simulink model "sampleModel6"  (Simulink 9.1)
settings: Solver=VariableStepAuto  StartTime=0.0  StopTime=10.0  RelTol=1e-3
undefined symbols (not defined in the file): DiscIntNeverNeededParam, Newton, Raphson
libraries: simulink x14
settings Model: Creator=DELL  LastModifiedBy=DELL
settings DataIOCC: SaveFormat=Dataset
settings OptimizationCC: LifeSpan=auto
settings DebuggingCC: UnderspecifiedInitializationDetection=Simplified  MergeDetectMultiDrivingBlocksExec=error  SFUnexpectedBacktrackingDiag=error  SFNoUnconditionalDefaultTransitionDiag=error  SFExecutionAtInitializationDiag=warning
settings HardwareCC: ProdBitPerPointer=64  ProdBitPerSizeT=64  ProdBitPerPtrDiffT=64  ProdLargestAtomicFloat=Float  ProdIntDivRoundTo=Zero  ProdEndianess=LittleEndian  ProdWordSize=64  ProdHWDeviceType=Intel->x86-64 (Windows64)
settings ModelReferenceCC: PropagateSignalLabelsOutOfModel=on
settings CodeAppCC: StateflowObjectComments=off
settings GRTTargetCC: TargetLangStandard=C99 (ISO)  CombineOutputUpdateFcns=on  GRTInterface=off
settings ConfigComp: CovMetricSettings=dwe  CovHtmlReporting=off  CovSaveCumulativeToWorkspaceVar=off  CovSaveSingleToWorkspaceVar=off  CovExternalEMLEnable=on

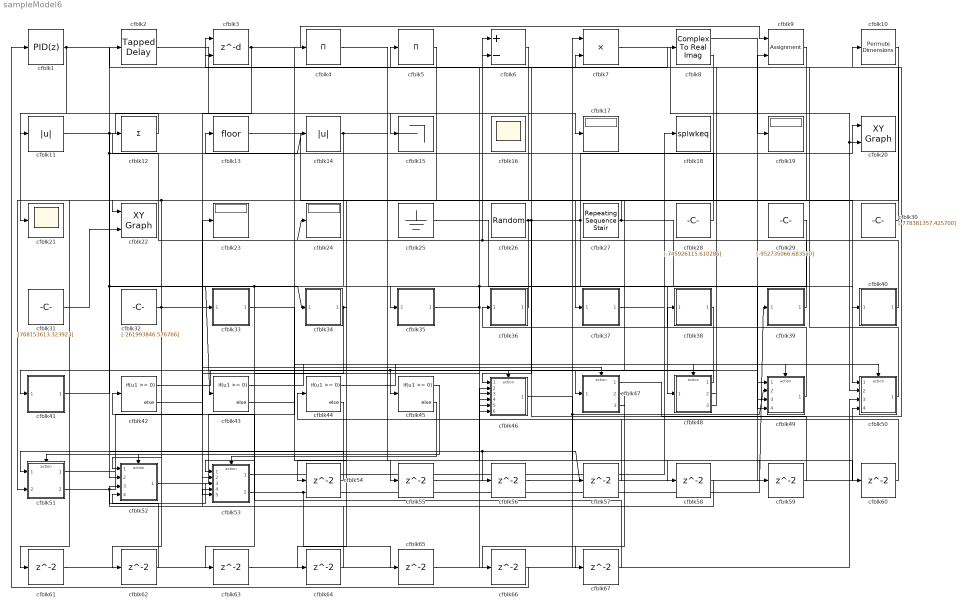
== system sampleModel6 ==
  cfblk1 : simulink/Continuous/PID Controller  Controller=PID  TimeDomain=Discrete-time  SampleTime=1  IntegratorMethod=Forward Euler  FilterMethod=Forward Euler  Form=Parallel  UseFilter=on  ControllerParametersSource=internal  P=1  I=1  D=0  N=100  InitialConditionSource=internal  InitialConditionForIntegrator=0  InitialConditionForFilter=0  ExternalReset=none  LimitOutput=off  UpperSaturationLimit=inf  LowerSaturationLimit=-inf  LinearizeAsGain=off  AntiWindupMode=none  Kb=1  TrackingMode=off  Kt=1  PParamMin=[]  PParamMax=[]  IParamMin=[]  IParamMax=[]  DParamMin=[]  DParamMax=[]  NParamMin=[]  NParamMax=[]  KbParamMin=[]  KbParamMax=[]  KtParamMin=[]  KtParamMax=[]  POutMin=[]  POutMax=[]  IOutMin=[]  IOutMax=[]  DOutMin=[]  DOutMax=[]  NOutMin=[]  NOutMax=[]  KbOutMin=[]  KbOutMax=[]  KtOutMin=[]  KtOutMax=[]  IntegratorOutMin=[]  IntegratorOutMax=[]  FilterOutMin=[]  FilterOutMax=[]  SumOutMin=[]  SumOutMax=[]  SumI1OutMin=[]  SumI1OutMax=[]  SumI2OutMin=[]  SumI2OutMax=[]  SumI3OutMin=[]  SumI3OutMax=[]  SumDOutMin=[]  SumDOutMax=[]  SaturationOutMin=[]  SaturationOutMax=[]  IntegratorContinuousStateAttributes=''  IntegratorStateMustResolveToSignalObject=off  IntegratorRTWStateStorageClass=Auto  FilterContinuousStateAttributes=''  FilterStateMustResolveToSignalObject=off  FilterRTWStateStorageClass=Auto  DifferentiatorICPrevScaledInput=0  DifferentiatorOutMin=[]  DifferentiatorOutMax=[]  FilterDiffOutCoefMin=[]  FilterDiffOutCoefMax=[]  SumDenOutMin=[]  SumDenOutMax=[]  SumNumOutMin=[]  SumNumOutMax=[]  ReciprocalOutMin=[]  ReciprocalOutMax=[]  DivideOutMin=[]  DivideOutMax=[]  TunerSelectOption=Transfer Function Based (PID Tuner App)
  cfblk10 : PermuteDimensions
  cfblk11 : Abs
  cfblk12 : Sum  Inputs=+
  cfblk13 : Rounding
  cfblk14 : Abs
  cfblk15 : Terminator
  cfblk16 : Scope
      settings: Floating=on
  cfblk{17,19,23..24} (4 alike) : Display
  cfblk18 : ToWorkspace  VariableName=splwkeq  SaveFormat=Timeseries  SampleTime=-1
  cfblk2 : simulink/Discrete/Tapped Delay  vinit=0.0  samptime=-1  NumDelays=1  DelayOrder=Oldest  includeCurrent=off
  cfblk20 : simulink/Sinks/XY Graph  xmin=-1  xmax=1  ymin=-1  ymax=1  st=-1
  cfblk21 : Scope
  cfblk22 : simulink/Sinks/XY Graph  xmin=-1  xmax=1  ymin=-1  ymax=1  st=-1
  cfblk25 : Ground
  cfblk26 : UniformRandomNumber  Minimum=[-3759994456.876560]  Maximum=[3279415969.732488]  Seed=[80296531.000000]  SampleTime=0.1
  cfblk27 : simulink/Sources/Repeating Sequence Stair  OutValues=[998955717.271784, 961956321.864293]  tsamp=-1  OutMin=[]  OutMax=[]  OutDataTypeStr=double  OutputDataTypeScalingMode=double  OutDataType=fixdt(0,8)  ConRadixGroup=Best Precision: Vector-wise  OutScaling=2^-12
  cfblk28 : Constant  Value=[-745926115.610286]  SampleTime=1
  cfblk29 : Constant  Value=[-952735066.683550]  SampleTime=1
  cfblk3 : Delay  DelayLengthSource=Input port  SampleTime=1
      settings: InputPortMap=u0,p1
  cfblk30 : Constant  Value=[-778381357.425700]  SampleTime=1
  cfblk31 : Constant  Value=[768153613.323923]  SampleTime=1
  cfblk32 : Constant  Value=[-261993846.576766]  SampleTime=1
  cfblk33 : Subsystem
  cfblk34 : Subsystem
  cfblk35 : Subsystem
  cfblk36 : Subsystem
  cfblk37 : Subsystem
  cfblk38 : Subsystem
  cfblk39 : Subsystem
  cfblk4 : Product  Inputs=*
  cfblk40 : Subsystem
  cfblk41 : Subsystem
  cfblk{42..45} (4 alike) : If  IfExpression=u1 >= 0  SampleTime=1
  cfblk46 : Subsystem  TreatAsAtomicUnit=on
  cfblk47 : Subsystem  TreatAsAtomicUnit=on
  cfblk48 : Subsystem  TreatAsAtomicUnit=on
  cfblk49 : Subsystem  TreatAsAtomicUnit=on
  cfblk5 : Product  Inputs=*
  cfblk50 : Subsystem  TreatAsAtomicUnit=on
  cfblk51 : Subsystem  TreatAsAtomicUnit=on
  cfblk52 : Subsystem  TreatAsAtomicUnit=on
  cfblk53 : Subsystem  TreatAsAtomicUnit=on
  cfblk{54..67} (14 alike) : Delay  SampleTime=1
  cfblk6 : Sum  Inputs=+-
  cfblk7 : Product  Inputs=**
  cfblk8 : ComplexToRealImag
  cfblk9 : Assignment  DiagnosticForDimensions=Warning  IndexOptions=Index vector (dialog)  Indices=1  OutputSizes=1
  wires:
  cfblk28/1 -> cfblk13/1
  cfblk49/1(cfblk2) -> cfblk36/1(cfblk1)
  cfblk27/1 -> cfblk22/1, cfblk49/4(cfblk9)
  cfblk29/1 -> cfblk43/1, cfblk46/5(cfblk12)
  cfblk26/1 -> cfblk48/1(cfblk1), cfblk20/1, cfblk46/1(cfblk1), cfblk46/6(cfblk13)
  cfblk31/1 -> cfblk22/2
  cfblk3/1 -> cfblk9/1, cfblk53/5(cfblk10)
  cfblk50/1(cfblk2) -> cfblk3/1
  cfblk47/1(cfblk2) -> cfblk10/1
  cfblk48/1(cfblk2) -> cfblk41/1(cfblk1)
  cfblk53/1(cfblk2) -> cfblk18/1
  cfblk48/2(cfblk8) -> cfblk38/1(cfblk1)
  cfblk1/1 -> cfblk21/1, cfblk7/2
  cfblk10/1 -> cfblk37/1(cfblk1)
  cfblk40/1(cfblk2) -> cfblk24/1, cfblk6/2
  cfblk36/1(cfblk2) -> cfblk35/1(cfblk1)
  cfblk11/1 -> cfblk56/1, cfblk57/1, cfblk34/1(cfblk1), cfblk17/1
  cfblk2/1 -> cfblk15/1
  cfblk53/2(cfblk11) -> cfblk39/1(cfblk1), cfblk65/1
  cfblk13/1 -> cfblk50/1(cfblk1)
  cfblk48/3(cfblk9) -> cfblk6/1
  cfblk30/1 -> cfblk5/1
  cfblk37/1(cfblk2) -> cfblk40/1(cfblk1)
  cfblk38/1(cfblk2) -> cfblk45/1, cfblk53/2(cfblk7)
  cfblk8/1 -> cfblk19/1
  cfblk9/1 -> cfblk47/1(cfblk1)
  cfblk52/1(cfblk2) -> cfblk4/1
  cfblk41/1(cfblk2) -> cfblk2/1, cfblk14/1
  cfblk5/1 -> cfblk51/2(cfblk14)
  cfblk51/1(cfblk2) -> cfblk33/1(cfblk1)
  cfblk39/1(cfblk2) -> cfblk12/1
  cfblk35/1(cfblk2) -> cfblk8/1, cfblk60/1
  cfblk7/1 -> cfblk50/2(cfblk10), cfblk20/2
  cfblk51/2(cfblk15) -> cfblk23/1, cfblk53/3(cfblk8)
  cfblk25/1 -> cfblk49/1(cfblk1)
  cfblk12/1 -> cfblk11/1
  cfblk32/1 -> cfblk52/1(cfblk1), cfblk46/3(cfblk10)
  cfblk8/2 -> cfblk61/1, cfblk62/1
  cfblk14/1 -> cfblk52/2(cfblk13), cfblk53/1(cfblk1), cfblk49/3(cfblk8)
  cfblk46/1(cfblk2) -> cfblk49/2(cfblk7), cfblk58/1
  cfblk34/1(cfblk2) -> cfblk63/1, cfblk64/1
  cfblk42/1 -> cfblk46/Action
  cfblk42/2 -> cfblk47/Action
  cfblk43/1 -> cfblk48/Action
  cfblk43/2 -> cfblk49/Action
  cfblk44/1 -> cfblk50/Action
  cfblk44/2 -> cfblk51/Action
  cfblk45/1 -> cfblk52/Action
  cfblk45/2 -> cfblk53/Action
  cfblk6/1 -> cfblk54/1
  cfblk54/1 -> cfblk51/1(cfblk1)
  cfblk33/1(cfblk2) -> cfblk55/1
  cfblk55/1 -> cfblk9/2
  cfblk56/1 -> cfblk50/4(cfblk12)
  cfblk57/1 -> cfblk46/2(cfblk9)
  cfblk58/1 -> cfblk52/3(cfblk14)
  cfblk4/1 -> cfblk59/1
  cfblk59/1 -> cfblk3/2
  cfblk60/1 -> cfblk44/1
  cfblk61/1 -> cfblk50/3(cfblk11)
  cfblk62/1 -> cfblk52/4(cfblk15)
  cfblk63/1 -> cfblk7/1
  cfblk64/1 -> cfblk53/4(cfblk9)
  cfblk65/1 -> cfblk46/4(cfblk11)
  cfblk47/2(cfblk13) -> cfblk66/1
  cfblk66/1 -> cfblk1/1
  cfblk47/3(cfblk14) -> cfblk67/1
  cfblk67/1 -> cfblk42/1

== system sampleModel6/cfblk33 ==
  cfblk1 : Inport
  cfblk2 : Outport
  wires:
  cfblk1/1 -> cfblk2/1

== system sampleModel6/cfblk34 ==
  cfblk1 : Inport
  cfblk2 : Outport
  wires:
  cfblk1/1 -> cfblk2/1

== system sampleModel6/cfblk35 ==
  cfblk1 : Inport
  cfblk2 : Outport
  wires:
  cfblk1/1 -> cfblk2/1

== system sampleModel6/cfblk36 ==
  cfblk1 : Inport
  cfblk2 : Outport
  wires:
  cfblk1/1 -> cfblk2/1

== system sampleModel6/cfblk37 ==
  cfblk1 : Inport
  cfblk2 : Outport
  wires:
  cfblk1/1 -> cfblk2/1

== system sampleModel6/cfblk38 ==
  cfblk1 : Inport
  cfblk2 : Outport
  wires:
  cfblk1/1 -> cfblk2/1

== system sampleModel6/cfblk39 ==
  cfblk1 : Inport
  cfblk2 : Outport
  wires:
  cfblk1/1 -> cfblk2/1

== system sampleModel6/cfblk40 ==
  cfblk1 : Inport
  cfblk2 : Outport
  wires:
  cfblk1/1 -> cfblk2/1

== system sampleModel6/cfblk41 ==
  cfblk1 : Inport
  cfblk2 : Outport
  wires:
  cfblk1/1 -> cfblk2/1

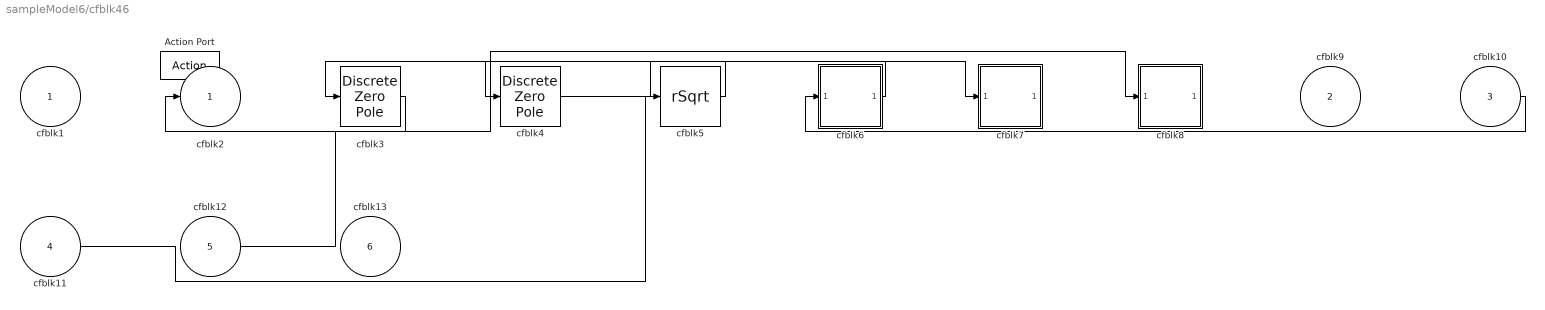
== system sampleModel6/cfblk46 ==
  cfblk1 : Inport
  cfblk9 : Inport  Port=2
  cfblk10 : Inport  Port=3
  cfblk11 : Inport  Port=4
  cfblk12 : Inport  Port=5
  cfblk13 : Inport  Port=6
  Action Port : ActionPort  ActionType=then
  cfblk3 : DiscreteZeroPole  Poles=[0 0.5]  Gain=1  SampleTime=-1
  cfblk4 : DiscreteZeroPole  Poles=[0 0.5]  Gain=1  SampleTime=-1
  cfblk5 : Sqrt  Operator=rSqrt  AlgorithmType=Newton-Raphson  SaturateOnIntegerOverflow=on
  cfblk6 : Subsystem
  cfblk7 : Subsystem
  cfblk8 : Subsystem
  cfblk2 : Outport
  wires:
  cfblk4/1 -> cfblk7/1(cfblk1)
  cfblk10/1 -> cfblk6/1(cfblk1)
  cfblk12/1 -> cfblk8/1(cfblk1)
  cfblk6/1(cfblk2) -> cfblk3/1
  cfblk5/1 -> cfblk4/1
  cfblk11/1 -> cfblk5/1
  cfblk3/1 -> cfblk2/1

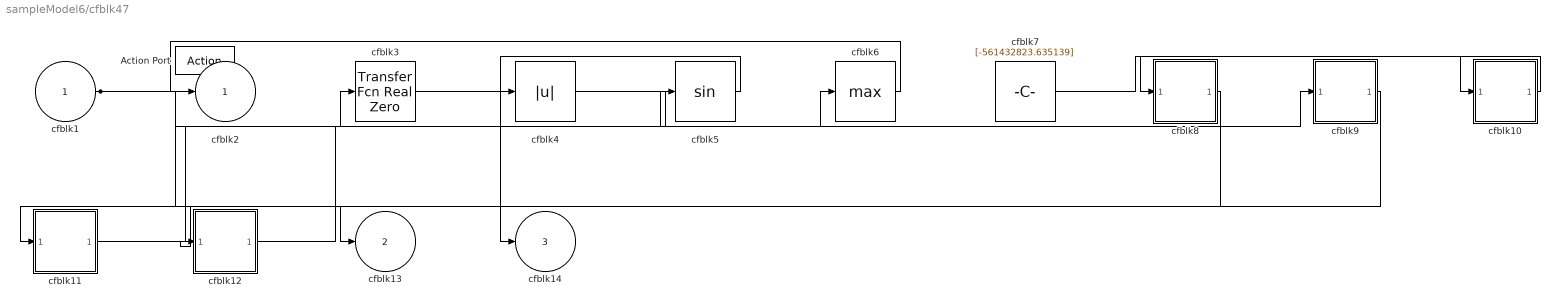
== system sampleModel6/cfblk47 ==
  cfblk1 : Inport
  Action Port : ActionPort  ActionType=else
  cfblk10 : Subsystem
  cfblk11 : Subsystem
  cfblk12 : Subsystem
  cfblk3 : simulink/Discrete/Transfer Fcn Real Zero  ZeroZ=0.75  ICPrevInput=0.0  DoSatur=off
      settings: SourceProductName=Simulink  SourceProductBaseCode=SL
  cfblk4 : Abs
  cfblk5 : Trigonometry
  cfblk6 : MinMax  Function=max
  cfblk7 : Constant  Value=[-561432823.635139]  SampleTime=1
  cfblk8 : Subsystem
  cfblk9 : Subsystem
  cfblk2 : Outport
  cfblk13 : Outport  Port=2
  cfblk14 : Outport  Port=3
  wires:
  cfblk11/1(cfblk2) -> cfblk3/1
  cfblk6/1 -> cfblk2/1
  cfblk9/1(cfblk2) -> cfblk12/1(cfblk1)
  cfblk10/1(cfblk2) -> cfblk8/1(cfblk1)
  cfblk3/1 -> cfblk14/1
  cfblk5/1 -> cfblk4/1
  cfblk4/1 -> cfblk9/1(cfblk1)
  cfblk1/1 -> cfblk13/1, cfblk5/1
  cfblk7/1 -> cfblk10/1(cfblk1)
  cfblk8/1(cfblk2) -> cfblk11/1(cfblk1)
  cfblk12/1(cfblk2) -> cfblk6/1

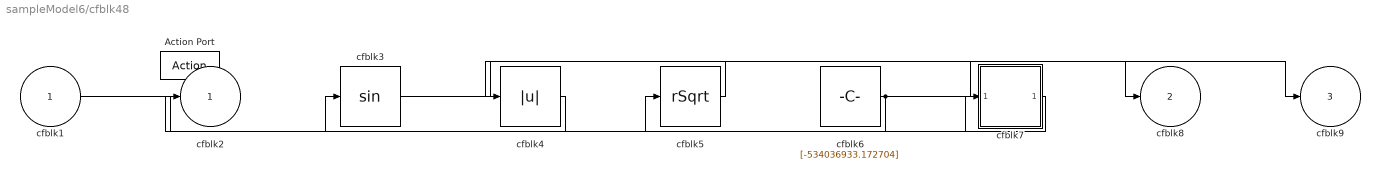
== system sampleModel6/cfblk48 ==
  cfblk1 : Inport
  Action Port : ActionPort  ActionType=then
  cfblk3 : Trigonometry
  cfblk4 : Abs
  cfblk5 : Sqrt  Operator=rSqrt  AlgorithmType=Newton-Raphson  SaturateOnIntegerOverflow=on
  cfblk6 : Constant  Value=[-534036933.172704]  SampleTime=1
  cfblk7 : Subsystem
  cfblk2 : Outport
  cfblk8 : Outport  Port=2
  cfblk9 : Outport  Port=3
  wires:
  cfblk3/1 -> cfblk8/1
  cfblk4/1 -> cfblk3/1
  cfblk7/1(cfblk2) -> cfblk5/1
  cfblk5/1 -> cfblk4/1
  cfblk6/1 -> cfblk9/1, cfblk2/1
  cfblk1/1 -> cfblk7/1(cfblk1)

== system sampleModel6/cfblk49 ==
  cfblk1 : Inport
  cfblk7 : Inport  Port=2
  cfblk8 : Inport  Port=3
  cfblk9 : Inport  Port=4
  Action Port : ActionPort  ActionType=else
  cfblk3 : simulink/Continuous/PID Controller  Controller=PID  TimeDomain=Discrete-time  SampleTime=-1  IntegratorMethod=Forward Euler  FilterMethod=Forward Euler  Form=Parallel  UseFilter=on  ControllerParametersSource=internal  P=1  I=1  D=0  N=100  InitialConditionSource=internal  InitialConditionForIntegrator=0  InitialConditionForFilter=0  ExternalReset=none  LimitOutput=off  UpperSaturationLimit=inf  LowerSaturationLimit=-inf  LinearizeAsGain=off  AntiWindupMode=none  Kb=1  TrackingMode=off  Kt=1  PParamMin=[]  PParamMax=[]  IParamMin=[]  IParamMax=[]  DParamMin=[]  DParamMax=[]  NParamMin=[]  NParamMax=[]  KbParamMin=[]  KbParamMax=[]  KtParamMin=[]  KtParamMax=[]  POutMin=[]  POutMax=[]  IOutMin=[]  IOutMax=[]  DOutMin=[]  DOutMax=[]  NOutMin=[]  NOutMax=[]  KbOutMin=[]  KbOutMax=[]  KtOutMin=[]  KtOutMax=[]  IntegratorOutMin=[]  IntegratorOutMax=[]  FilterOutMin=[]  FilterOutMax=[]  SumOutMin=[]  SumOutMax=[]  SumI1OutMin=[]  SumI1OutMax=[]  SumI2OutMin=[]  SumI2OutMax=[]  SumI3OutMin=[]  SumI3OutMax=[]  SumDOutMin=[]  SumDOutMax=[]  SaturationOutMin=[]  SaturationOutMax=[]  IntegratorContinuousStateAttributes=''  IntegratorStateMustResolveToSignalObject=off  IntegratorRTWStateStorageClass=Auto  FilterContinuousStateAttributes=''  FilterStateMustResolveToSignalObject=off  FilterRTWStateStorageClass=Auto  DifferentiatorICPrevScaledInput=0  DifferentiatorOutMin=[]  DifferentiatorOutMax=[]  FilterDiffOutCoefMin=[]  FilterDiffOutCoefMax=[]  SumDenOutMin=[]  SumDenOutMax=[]  SumNumOutMin=[]  SumNumOutMax=[]  ReciprocalOutMin=[]  ReciprocalOutMax=[]  DivideOutMin=[]  DivideOutMax=[]  TunerSelectOption=Transfer Function Based (PID Tuner App)
  cfblk4 : simulink/Math Operations/MinMax Running Resettable  Function=min  vinit=0.0
  cfblk5 : Constant  Value=[144478436.825369]  SampleTime=1
  cfblk6 : Subsystem
  cfblk2 : Outport
  wires:
  cfblk9/1 -> cfblk3/1
  cfblk8/1 -> cfblk4/1
  cfblk5/1 -> cfblk2/1
  cfblk7/1 -> cfblk6/1(cfblk1)
  cfblk3/1 -> cfblk4/2

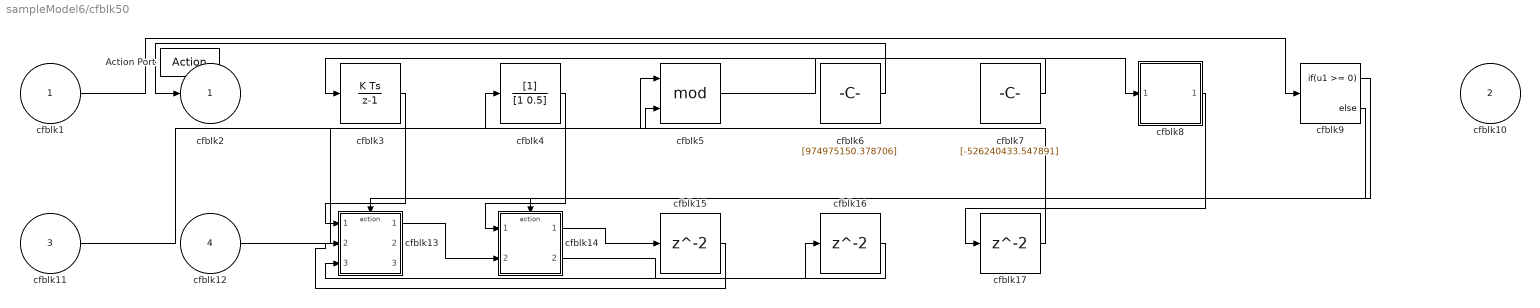
== system sampleModel6/cfblk50 ==
  cfblk1 : Inport
  cfblk10 : Inport  Port=2
  cfblk11 : Inport  Port=3
  cfblk12 : Inport  Port=4
  Action Port : ActionPort  ActionType=then
  cfblk13 : Subsystem  TreatAsAtomicUnit=on
  cfblk14 : Subsystem  TreatAsAtomicUnit=on
  cfblk15 : Delay
  cfblk16 : Delay
  cfblk17 : Delay
  cfblk3 : DiscreteIntegrator  SampleTime=-1  ICPrevOutput=DiscIntNeverNeededParam  ICPrevScaledInput=DiscIntNeverNeededParam
  cfblk4 : DiscreteFilter
  cfblk5 : Math  Operator=mod  SaturateOnIntegerOverflow=on
  cfblk6 : Constant  Value=[974975150.378706]  SampleTime=1
  cfblk7 : Constant  Value=[-526240433.547891]  SampleTime=1
  cfblk8 : Subsystem
  cfblk9 : If  IfExpression=u1 >= 0  SampleTime=1
  cfblk2 : Outport
  wires:
  cfblk4/1 -> cfblk14/1(cfblk1)
  cfblk6/1 -> cfblk2/1
  cfblk12/1 -> cfblk5/2
  cfblk7/1 -> cfblk3/1
  cfblk5/1 -> cfblk8/1(cfblk1)
  cfblk11/1 -> cfblk4/1
  cfblk1/1 -> cfblk9/1
  cfblk3/1 -> cfblk13/1(cfblk1)
  cfblk13/1(cfblk2) -> cfblk14/2(cfblk14)
  cfblk9/1 -> cfblk13/Action
  cfblk9/2 -> cfblk14/Action
  cfblk14/1(cfblk2) -> cfblk15/1
  cfblk15/1 -> cfblk13/2(cfblk13)
  cfblk14/2(cfblk15) -> cfblk16/1
  cfblk16/1 -> cfblk13/3(cfblk14)
  cfblk8/1(cfblk2) -> cfblk17/1
  cfblk17/1 -> cfblk5/1

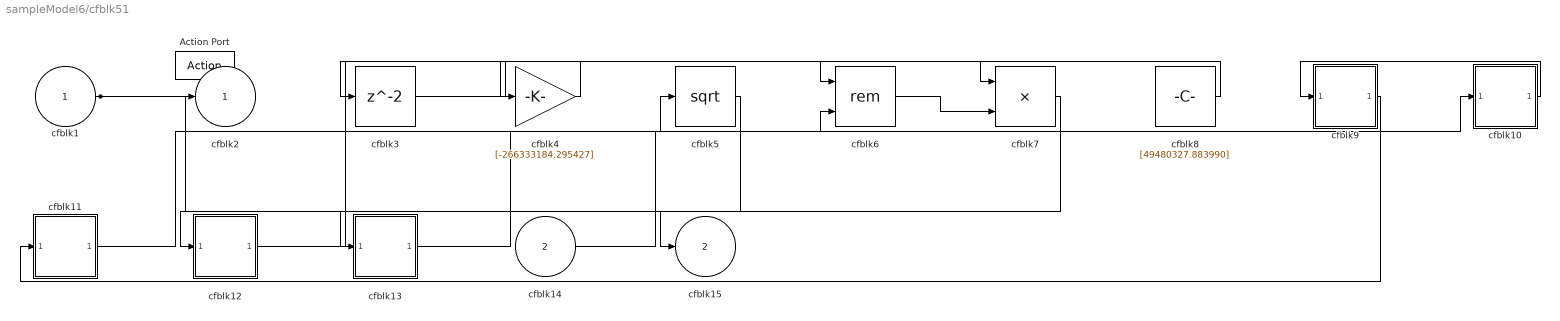
== system sampleModel6/cfblk51 ==
  cfblk1 : Inport
  cfblk14 : Inport  Port=2
  Action Port : ActionPort  ActionType=else
  cfblk10 : Subsystem
  cfblk11 : Subsystem
  cfblk12 : Subsystem
  cfblk13 : Subsystem
  cfblk3 : Delay
  cfblk4 : Gain  Gain=[-266333184.295427]
  cfblk5 : Sqrt  SaturateOnIntegerOverflow=on
  cfblk6 : Math  Operator=rem  SaturateOnIntegerOverflow=on
  cfblk7 : Product
  cfblk8 : Constant  Value=[49480327.883990]  SampleTime=1
  cfblk9 : Subsystem
  cfblk2 : Outport
  cfblk15 : Outport  Port=2
  wires:
  cfblk13/1(cfblk2) -> cfblk5/1
  cfblk12/1(cfblk2) -> cfblk7/1
  cfblk4/1 -> cfblk3/1
  cfblk1/1 -> cfblk13/1(cfblk1), cfblk2/1
  cfblk9/1(cfblk2) -> cfblk11/1(cfblk1)
  cfblk6/1 -> cfblk7/2
  cfblk7/1 -> cfblk15/1
  cfblk3/1 -> cfblk6/1
  cfblk8/1 -> cfblk4/1
  cfblk5/1 -> cfblk12/1(cfblk1)
  cfblk11/1(cfblk2) -> cfblk6/2
  cfblk14/1 -> cfblk10/1(cfblk1)
  cfblk10/1(cfblk2) -> cfblk9/1(cfblk1)

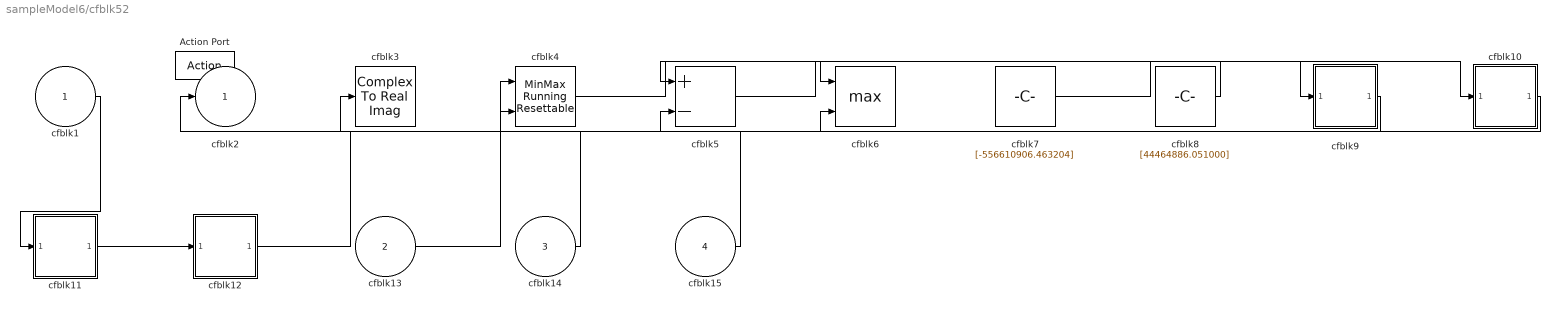
== system sampleModel6/cfblk52 ==
  cfblk1 : Inport
  cfblk13 : Inport  Port=2
  cfblk14 : Inport  Port=3
  cfblk15 : Inport  Port=4
  Action Port : ActionPort  ActionType=then
  cfblk10 : Subsystem
  cfblk11 : Subsystem
  cfblk12 : Subsystem
  cfblk3 : ComplexToRealImag
  cfblk4 : simulink/Math Operations/MinMax Running Resettable  Function=min  vinit=0.0
  cfblk5 : Sum  Inputs=+-
  cfblk6 : MinMax  Function=max  Inputs=2
  cfblk7 : Constant  Value=[-556610906.463204]  SampleTime=1
  cfblk8 : Constant  Value=[44464886.051000]  SampleTime=1
  cfblk9 : Subsystem
  cfblk2 : Outport
  wires:
  cfblk7/1 -> cfblk10/1(cfblk1)
  cfblk10/1(cfblk2) -> cfblk2/1
  cfblk13/1 -> cfblk4/1
  cfblk4/1 -> cfblk6/1
  cfblk11/1(cfblk2) -> cfblk12/1(cfblk1)
  cfblk1/1 -> cfblk11/1(cfblk1)
  cfblk14/1 -> cfblk3/1
  cfblk12/1(cfblk2) -> cfblk6/2
  cfblk8/1 -> cfblk5/1
  cfblk15/1 -> cfblk5/2
  cfblk5/1 -> cfblk9/1(cfblk1)
  cfblk9/1(cfblk2) -> cfblk4/2

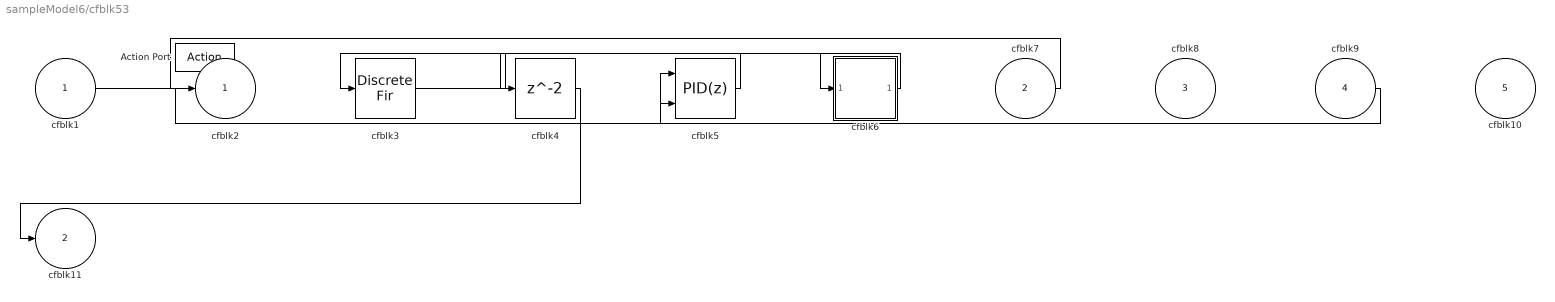
== system sampleModel6/cfblk53 ==
  cfblk1 : Inport
  cfblk7 : Inport  Port=2
  cfblk8 : Inport  Port=3
  cfblk9 : Inport  Port=4
  cfblk10 : Inport  Port=5
  Action Port : ActionPort  ActionType=else
  cfblk3 : DiscreteFir
  cfblk4 : Delay
  cfblk5 : simulink/Continuous/PID Controller (2DOF)  Controller=PID  TimeDomain=Discrete-time  SampleTime=-1  IntegratorMethod=Forward Euler  FilterMethod=Forward Euler  Form=Parallel  UseFilter=on  ControllerParametersSource=internal  P=1  I=1  D=0  N=100  b=1  c=1  InitialConditionSource=internal  InitialConditionForIntegrator=0  InitialConditionForFilter=0  ExternalReset=none  LimitOutput=off  UpperSaturationLimit=inf  LowerSaturationLimit=-inf  LinearizeAsGain=off  AntiWindupMode=none  Kb=1  TrackingMode=off  Kt=1  PParamMin=[]  PParamMax=[]  IParamMin=[]  IParamMax=[]  DParamMin=[]  DParamMax=[]  NParamMin=[]  NParamMax=[]  bParamMin=[]  bParamMax=[]  cParamMin=[]  cParamMax=[]  KbParamMin=[]  KbParamMax=[]  KtParamMin=[]  KtParamMax=[]  POutMin=[]  POutMax=[]  IOutMin=[]  IOutMax=[]  DOutMin=[]  DOutMax=[]  NOutMin=[]  NOutMax=[]  bOutMin=[]  bOutMax=[]  cOutMin=[]  cOutMax=[]  KbOutMin=[]  KbOutMax=[]  KtOutMin=[]  KtOutMax=[]  IntegratorOutMin=[]  IntegratorOutMax=[]  FilterOutMin=[]  FilterOutMax=[]  SumOutMin=[]  SumOutMax=[]  Sum1OutMin=[]  Sum1OutMax=[]  Sum2OutMin=[]  Sum2OutMax=[]  Sum3OutMin=[]  Sum3OutMax=[]  SumI1OutMin=[]  SumI1OutMax=[]  SumI2OutMin=[]  SumI2OutMax=[]  SumI3OutMin=[]  SumI3OutMax=[]  SumDOutMin=[]  SumDOutMax=[]  SaturationOutMin=[]  SaturationOutMax=[]  IntegratorContinuousStateAttributes=''  IntegratorStateMustResolveToSignalObject=off  IntegratorRTWStateStorageClass=Auto  FilterContinuousStateAttributes=''  FilterStateMustResolveToSignalObject=off  FilterRTWStateStorageClass=Auto  DifferentiatorICPrevScaledInput=0  DifferentiatorOutMin=[]  DifferentiatorOutMax=[]  FilterDiffOutCoefMin=[]  FilterDiffOutCoefMax=[]  SumDenOutMin=[]  SumDenOutMax=[]  SumNumOutMin=[]  SumNumOutMax=[]  ReciprocalOutMin=[]  ReciprocalOutMax=[]  DivideOutMin=[]  DivideOutMax=[]  TunerSelectOption=Transfer Function Based (PID Tuner App)
  cfblk6 : Subsystem
  cfblk2 : Outport
  cfblk11 : Outport  Port=2
  wires:
  cfblk5/1 -> cfblk3/1
  cfblk4/1 -> cfblk11/1
  cfblk7/1 -> cfblk2/1
  cfblk3/1 -> cfblk6/1(cfblk1)
  cfblk9/1 -> cfblk5/1
  cfblk6/1(cfblk2) -> cfblk4/1
  cfblk1/1 -> cfblk5/2

== system sampleModel6/cfblk46/cfblk6 ==
  cfblk1 : Inport
  cfblk2 : Outport
  wires:
  cfblk1/1 -> cfblk2/1

== system sampleModel6/cfblk46/cfblk7 ==
  cfblk1 : Inport
  cfblk2 : Outport
  wires:
  cfblk1/1 -> cfblk2/1

== system sampleModel6/cfblk46/cfblk8 ==
  cfblk1 : Inport
  cfblk2 : Outport
  wires:
  cfblk1/1 -> cfblk2/1

== system sampleModel6/cfblk47/cfblk10 ==
  cfblk1 : Inport
  cfblk2 : Outport
  wires:
  cfblk1/1 -> cfblk2/1

== system sampleModel6/cfblk47/cfblk11 ==
  cfblk1 : Inport
  cfblk2 : Outport
  wires:
  cfblk1/1 -> cfblk2/1

== system sampleModel6/cfblk47/cfblk12 ==
  cfblk1 : Inport
  cfblk2 : Outport
  wires:
  cfblk1/1 -> cfblk2/1

== system sampleModel6/cfblk47/cfblk8 ==
  cfblk1 : Inport
  cfblk2 : Outport
  wires:
  cfblk1/1 -> cfblk2/1

== system sampleModel6/cfblk47/cfblk9 ==
  cfblk1 : Inport
  cfblk2 : Outport
  wires:
  cfblk1/1 -> cfblk2/1

== system sampleModel6/cfblk48/cfblk7 ==
  cfblk1 : Inport
  cfblk2 : Outport
  wires:
  cfblk1/1 -> cfblk2/1

== system sampleModel6/cfblk49/cfblk6 ==
  cfblk1 : Inport
  cfblk2 : Outport
  wires:
  cfblk1/1 -> cfblk2/1

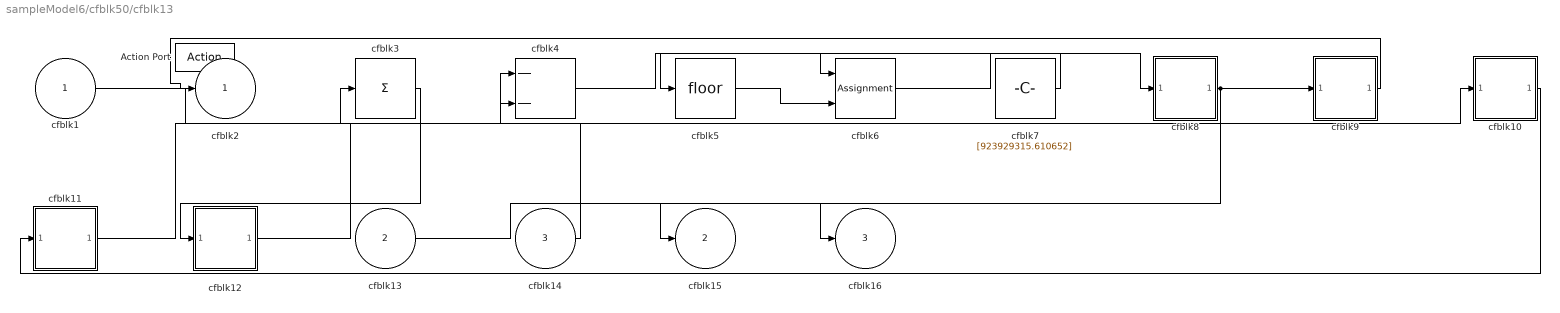
== system sampleModel6/cfblk50/cfblk13 ==
  cfblk1 : Inport
  cfblk13 : Inport  Port=2
  cfblk14 : Inport  Port=3
  Action Port : ActionPort  ActionType=then
  cfblk10 : Subsystem
  cfblk11 : Subsystem
  cfblk12 : Subsystem
  cfblk3 : Sum  Inputs=+
  cfblk4 : Sum  Inputs=--
  cfblk5 : Rounding
  cfblk6 : Assignment  DiagnosticForDimensions=Warning  IndexOptions=Index vector (dialog)  Indices=1  OutputSizes=1
  cfblk7 : Constant  Value=[923929315.610652]  SampleTime=1
  cfblk8 : Subsystem
  cfblk9 : Subsystem
  cfblk2 : Outport
  cfblk15 : Outport  Port=2
  cfblk16 : Outport  Port=3
  wires:
  cfblk1/1 -> cfblk10/1(cfblk1)
  cfblk7/1 -> cfblk5/1
  cfblk8/1(cfblk2) -> cfblk15/1, cfblk9/1(cfblk1)
  cfblk10/1(cfblk2) -> cfblk11/1(cfblk1)
  cfblk3/1 -> cfblk12/1(cfblk1)
  cfblk13/1 -> cfblk16/1
  cfblk9/1(cfblk2) -> cfblk2/1
  cfblk12/1(cfblk2) -> cfblk4/1
  cfblk11/1(cfblk2) -> cfblk4/2
  cfblk6/1 -> cfblk8/1(cfblk1)
  cfblk4/1 -> cfblk6/1
  cfblk5/1 -> cfblk6/2
  cfblk14/1 -> cfblk3/1

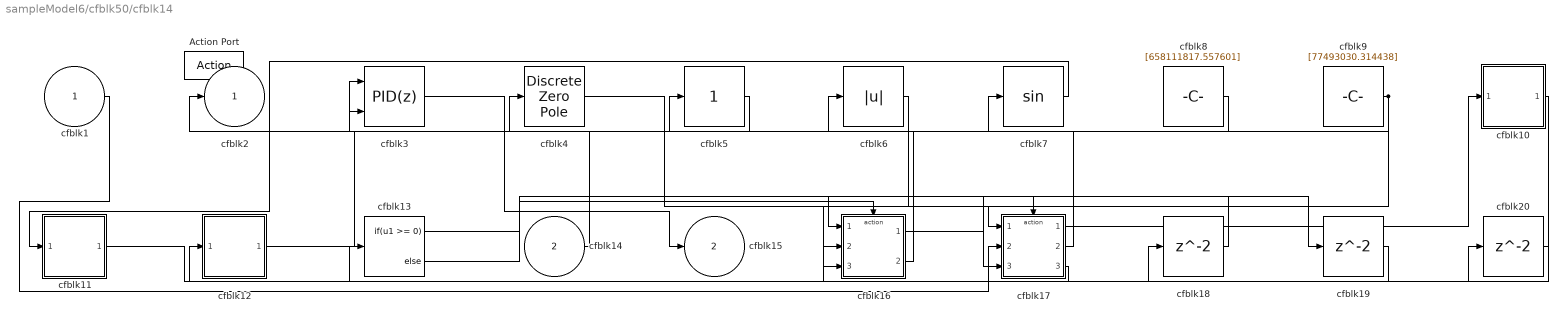
== system sampleModel6/cfblk50/cfblk14 ==
  cfblk1 : Inport
  cfblk14 : Inport  Port=2
  Action Port : ActionPort  ActionType=else
  cfblk10 : Subsystem
  cfblk11 : Subsystem
  cfblk12 : Subsystem
  cfblk13 : If  IfExpression=u1 >= 0  SampleTime=1
  cfblk16 : Subsystem  TreatAsAtomicUnit=on
  cfblk17 : Subsystem  TreatAsAtomicUnit=on
  cfblk18 : Delay
  cfblk19 : Delay
  cfblk20 : Delay
  cfblk3 : simulink/Continuous/PID Controller (2DOF)  Controller=PID  TimeDomain=Discrete-time  SampleTime=-1  IntegratorMethod=Forward Euler  FilterMethod=Forward Euler  Form=Parallel  UseFilter=on  ControllerParametersSource=internal  P=1  I=1  D=0  N=100  b=1  c=1  InitialConditionSource=internal  InitialConditionForIntegrator=0  InitialConditionForFilter=0  ExternalReset=none  LimitOutput=off  UpperSaturationLimit=inf  LowerSaturationLimit=-inf  LinearizeAsGain=off  AntiWindupMode=none  Kb=1  TrackingMode=off  Kt=1  PParamMin=[]  PParamMax=[]  IParamMin=[]  IParamMax=[]  DParamMin=[]  DParamMax=[]  NParamMin=[]  NParamMax=[]  bParamMin=[]  bParamMax=[]  cParamMin=[]  cParamMax=[]  KbParamMin=[]  KbParamMax=[]  KtParamMin=[]  KtParamMax=[]  POutMin=[]  POutMax=[]  IOutMin=[]  IOutMax=[]  DOutMin=[]  DOutMax=[]  NOutMin=[]  NOutMax=[]  bOutMin=[]  bOutMax=[]  cOutMin=[]  cOutMax=[]  KbOutMin=[]  KbOutMax=[]  KtOutMin=[]  KtOutMax=[]  IntegratorOutMin=[]  IntegratorOutMax=[]  FilterOutMin=[]  FilterOutMax=[]  SumOutMin=[]  SumOutMax=[]  Sum1OutMin=[]  Sum1OutMax=[]  Sum2OutMin=[]  Sum2OutMax=[]  Sum3OutMin=[]  Sum3OutMax=[]  SumI1OutMin=[]  SumI1OutMax=[]  SumI2OutMin=[]  SumI2OutMax=[]  SumI3OutMin=[]  SumI3OutMax=[]  SumDOutMin=[]  SumDOutMax=[]  SaturationOutMin=[]  SaturationOutMax=[]  IntegratorContinuousStateAttributes=''  IntegratorStateMustResolveToSignalObject=off  IntegratorRTWStateStorageClass=Auto  FilterContinuousStateAttributes=''  FilterStateMustResolveToSignalObject=off  FilterRTWStateStorageClass=Auto  DifferentiatorICPrevScaledInput=0  DifferentiatorOutMin=[]  DifferentiatorOutMax=[]  FilterDiffOutCoefMin=[]  FilterDiffOutCoefMax=[]  SumDenOutMin=[]  SumDenOutMax=[]  SumNumOutMin=[]  SumNumOutMax=[]  ReciprocalOutMin=[]  ReciprocalOutMax=[]  DivideOutMin=[]  DivideOutMax=[]  TunerSelectOption=Transfer Function Based (PID Tuner App)
  cfblk4 : DiscreteZeroPole  Poles=[0 0.5]  Gain=1  SampleTime=-1
  cfblk5 : simulink/Math Operations/Slider Gain  gain=1  low=0  high=2
  cfblk6 : Abs
  cfblk7 : Trigonometry
  cfblk8 : Constant  Value=[658111817.557601]  SampleTime=1
  cfblk9 : Constant  Value=[77493030.314438]  SampleTime=1
  cfblk2 : Outport
  cfblk15 : Outport  Port=2
  wires:
  cfblk12/1(cfblk2) -> cfblk5/1
  cfblk7/1 -> cfblk11/1(cfblk1)
  cfblk14/1 -> cfblk4/1
  cfblk17/1(cfblk2) -> cfblk10/1(cfblk1)
  cfblk8/1 -> cfblk6/1
  cfblk4/1 -> cfblk17/1(cfblk1)
  cfblk17/2(cfblk15) -> cfblk7/1
  cfblk5/1 -> cfblk2/1
  cfblk3/1 -> cfblk15/1
  cfblk1/1 -> cfblk17/2(cfblk13)
  cfblk6/1 -> cfblk16/3(cfblk13)
  cfblk17/3(cfblk16) -> cfblk12/1(cfblk1)
  cfblk9/1 -> cfblk17/3(cfblk14), cfblk3/2
  cfblk16/2(cfblk14) -> cfblk3/1
  cfblk13/1 -> cfblk16/Action
  cfblk13/2 -> cfblk17/Action
  cfblk10/1(cfblk2) -> cfblk18/1
  cfblk18/1 -> cfblk16/1(cfblk1)
  cfblk16/1(cfblk2) -> cfblk19/1
  cfblk19/1 -> cfblk13/1
  cfblk11/1(cfblk2) -> cfblk20/1
  cfblk20/1 -> cfblk16/2(cfblk12)

== system sampleModel6/cfblk50/cfblk8 ==
  cfblk1 : Inport
  cfblk2 : Outport
  wires:
  cfblk1/1 -> cfblk2/1

== system sampleModel6/cfblk51/cfblk10 ==
  cfblk1 : Inport
  cfblk2 : Outport
  wires:
  cfblk1/1 -> cfblk2/1

== system sampleModel6/cfblk51/cfblk11 ==
  cfblk1 : Inport
  cfblk2 : Outport
  wires:
  cfblk1/1 -> cfblk2/1

== system sampleModel6/cfblk51/cfblk12 ==
  cfblk1 : Inport
  cfblk2 : Outport
  wires:
  cfblk1/1 -> cfblk2/1

== system sampleModel6/cfblk51/cfblk13 ==
  cfblk1 : Inport
  cfblk2 : Outport
  wires:
  cfblk1/1 -> cfblk2/1

== system sampleModel6/cfblk51/cfblk9 ==
  cfblk1 : Inport
  cfblk2 : Outport
  wires:
  cfblk1/1 -> cfblk2/1

== system sampleModel6/cfblk52/cfblk10 ==
  cfblk1 : Inport
  cfblk2 : Outport
  wires:
  cfblk1/1 -> cfblk2/1

== system sampleModel6/cfblk52/cfblk11 ==
  cfblk1 : Inport
  cfblk2 : Outport
  wires:
  cfblk1/1 -> cfblk2/1

== system sampleModel6/cfblk52/cfblk12 ==
  cfblk1 : Inport
  cfblk2 : Outport
  wires:
  cfblk1/1 -> cfblk2/1

== system sampleModel6/cfblk52/cfblk9 ==
  cfblk1 : Inport
  cfblk2 : Outport
  wires:
  cfblk1/1 -> cfblk2/1

== system sampleModel6/cfblk53/cfblk6 ==
  cfblk1 : Inport
  cfblk2 : Outport
  wires:
  cfblk1/1 -> cfblk2/1

== system sampleModel6/cfblk50/cfblk13/cfblk10 ==
  cfblk1 : Inport
  cfblk2 : Outport
  wires:
  cfblk1/1 -> cfblk2/1

== system sampleModel6/cfblk50/cfblk13/cfblk11 ==
  cfblk1 : Inport
  cfblk2 : Outport
  wires:
  cfblk1/1 -> cfblk2/1

== system sampleModel6/cfblk50/cfblk13/cfblk12 ==
  cfblk1 : Inport
  cfblk2 : Outport
  wires:
  cfblk1/1 -> cfblk2/1

== system sampleModel6/cfblk50/cfblk13/cfblk8 ==
  cfblk1 : Inport
  cfblk2 : Outport
  wires:
  cfblk1/1 -> cfblk2/1

== system sampleModel6/cfblk50/cfblk13/cfblk9 ==
  cfblk1 : Inport
  cfblk2 : Outport
  wires:
  cfblk1/1 -> cfblk2/1

== system sampleModel6/cfblk50/cfblk14/cfblk10 ==
  cfblk1 : Inport
  cfblk2 : Outport
  wires:
  cfblk1/1 -> cfblk2/1

== system sampleModel6/cfblk50/cfblk14/cfblk11 ==
  cfblk1 : Inport
  cfblk2 : Outport
  wires:
  cfblk1/1 -> cfblk2/1

== system sampleModel6/cfblk50/cfblk14/cfblk12 ==
  cfblk1 : Inport
  cfblk2 : Outport
  wires:
  cfblk1/1 -> cfblk2/1

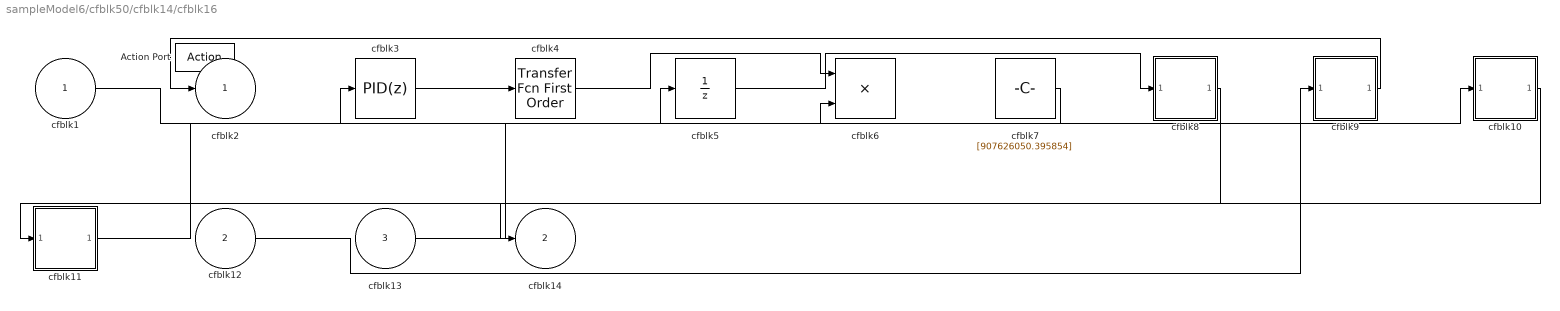
== system sampleModel6/cfblk50/cfblk14/cfblk16 ==
  cfblk1 : Inport
  cfblk12 : Inport  Port=2
  cfblk13 : Inport  Port=3
  Action Port : ActionPort  ActionType=then
  cfblk10 : Subsystem
  cfblk11 : Subsystem
  cfblk3 : simulink/Continuous/PID Controller  Controller=PID  TimeDomain=Discrete-time  SampleTime=-1  IntegratorMethod=Forward Euler  FilterMethod=Forward Euler  Form=Parallel  UseFilter=on  ControllerParametersSource=internal  P=1  I=1  D=0  N=100  InitialConditionSource=internal  InitialConditionForIntegrator=0  InitialConditionForFilter=0  ExternalReset=none  LimitOutput=off  UpperSaturationLimit=inf  LowerSaturationLimit=-inf  LinearizeAsGain=off  AntiWindupMode=none  Kb=1  TrackingMode=off  Kt=1  PParamMin=[]  PParamMax=[]  IParamMin=[]  IParamMax=[]  DParamMin=[]  DParamMax=[]  NParamMin=[]  NParamMax=[]  KbParamMin=[]  KbParamMax=[]  KtParamMin=[]  KtParamMax=[]  POutMin=[]  POutMax=[]  IOutMin=[]  IOutMax=[]  DOutMin=[]  DOutMax=[]  NOutMin=[]  NOutMax=[]  KbOutMin=[]  KbOutMax=[]  KtOutMin=[]  KtOutMax=[]  IntegratorOutMin=[]  IntegratorOutMax=[]  FilterOutMin=[]  FilterOutMax=[]  SumOutMin=[]  SumOutMax=[]  SumI1OutMin=[]  SumI1OutMax=[]  SumI2OutMin=[]  SumI2OutMax=[]  SumI3OutMin=[]  SumI3OutMax=[]  SumDOutMin=[]  SumDOutMax=[]  SaturationOutMin=[]  SaturationOutMax=[]  IntegratorContinuousStateAttributes=''  IntegratorStateMustResolveToSignalObject=off  IntegratorRTWStateStorageClass=Auto  FilterContinuousStateAttributes=''  FilterStateMustResolveToSignalObject=off  FilterRTWStateStorageClass=Auto  DifferentiatorICPrevScaledInput=0  DifferentiatorOutMin=[]  DifferentiatorOutMax=[]  FilterDiffOutCoefMin=[]  FilterDiffOutCoefMax=[]  SumDenOutMin=[]  SumDenOutMax=[]  SumNumOutMin=[]  SumNumOutMax=[]  ReciprocalOutMin=[]  ReciprocalOutMax=[]  DivideOutMin=[]  DivideOutMax=[]  TunerSelectOption=Transfer Function Based (PID Tuner App)
  cfblk4 : simulink/Discrete/Transfer Fcn First Order  PoleZ=0.95  ICPrevOutput=0.0  DoSatur=off
      settings: SourceProductName=Simulink
  cfblk5 : UnitDelay  SampleTime=-1
  cfblk6 : Product
  cfblk7 : Constant  Value=[907626050.395854]  SampleTime=1
  cfblk8 : Subsystem
  cfblk9 : Subsystem
  cfblk2 : Outport
  cfblk14 : Outport  Port=2
  wires:
  cfblk8/1(cfblk2) -> cfblk11/1(cfblk1)
  cfblk5/1 -> cfblk8/1(cfblk1)
  cfblk12/1 -> cfblk9/1(cfblk1)
  cfblk7/1 -> cfblk5/1
  cfblk3/1 -> cfblk4/1
  cfblk13/1 -> cfblk10/1(cfblk1)
  cfblk10/1(cfblk2) -> cfblk14/1
  cfblk9/1(cfblk2) -> cfblk2/1
  cfblk1/1 -> cfblk3/1
  cfblk4/1 -> cfblk6/1
  cfblk11/1(cfblk2) -> cfblk6/2

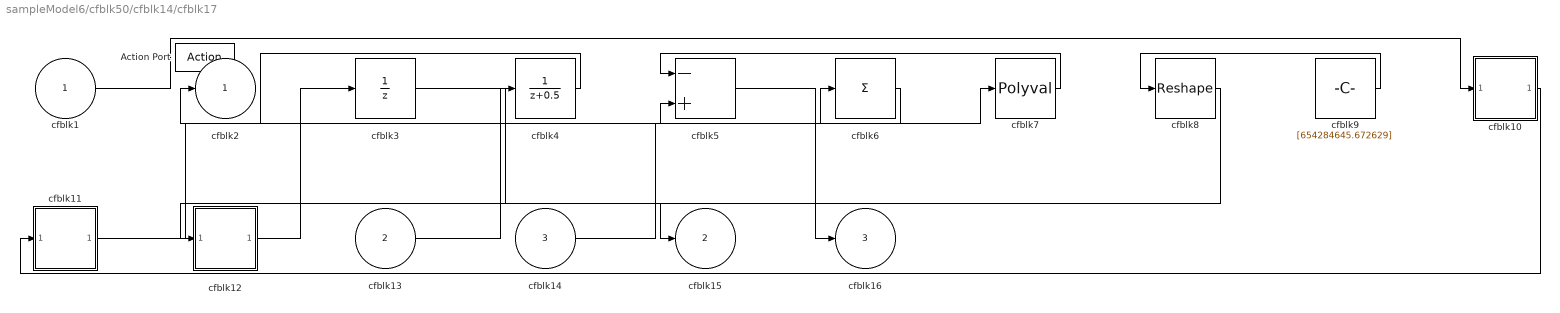
== system sampleModel6/cfblk50/cfblk14/cfblk17 ==
  cfblk1 : Inport
  cfblk13 : Inport  Port=2
  cfblk14 : Inport  Port=3
  Action Port : ActionPort  ActionType=else
  cfblk10 : Subsystem
  cfblk11 : Subsystem
  cfblk12 : Subsystem
  cfblk3 : UnitDelay  SampleTime=-1
  cfblk4 : DiscreteTransferFcn
  cfblk5 : Sum  Inputs=-+
  cfblk6 : Sum  Inputs=+
  cfblk7 : Polyval  Coefs=[ +2.081618890e-019, -1.441693666e-014, +4.719686976e-010, -8.536869453e-006, +1.621573104e-001, -8.087801117e+001 ]
  cfblk8 : Reshape
  cfblk9 : Constant  Value=[654284645.672629]  SampleTime=1
  cfblk2 : Outport
  cfblk15 : Outport  Port=2
  cfblk16 : Outport  Port=3
  wires:
  cfblk12/1(cfblk2) -> cfblk3/1
  cfblk1/1 -> cfblk10/1(cfblk1)
  cfblk4/1 -> cfblk2/1
  cfblk3/1 -> cfblk15/1
  cfblk7/1 -> cfblk5/1
  cfblk13/1 -> cfblk4/1
  cfblk10/1(cfblk2) -> cfblk11/1(cfblk1)
  cfblk9/1 -> cfblk8/1
  cfblk11/1(cfblk2) -> cfblk6/1
  cfblk6/1 -> cfblk5/2
  cfblk14/1 -> cfblk7/1
  cfblk5/1 -> cfblk16/1
  cfblk8/1 -> cfblk12/1(cfblk1)

== system sampleModel6/cfblk50/cfblk14/cfblk16/cfblk10 ==
  cfblk1 : Inport
  cfblk2 : Outport
  wires:
  cfblk1/1 -> cfblk2/1

== system sampleModel6/cfblk50/cfblk14/cfblk16/cfblk11 ==
  cfblk1 : Inport
  cfblk2 : Outport
  wires:
  cfblk1/1 -> cfblk2/1

== system sampleModel6/cfblk50/cfblk14/cfblk16/cfblk8 ==
  cfblk1 : Inport
  cfblk2 : Outport
  wires:
  cfblk1/1 -> cfblk2/1

== system sampleModel6/cfblk50/cfblk14/cfblk16/cfblk9 ==
  cfblk1 : Inport
  cfblk2 : Outport
  wires:
  cfblk1/1 -> cfblk2/1

== system sampleModel6/cfblk50/cfblk14/cfblk17/cfblk10 ==
  cfblk1 : Inport
  cfblk2 : Outport
  wires:
  cfblk1/1 -> cfblk2/1

== system sampleModel6/cfblk50/cfblk14/cfblk17/cfblk11 ==
  cfblk1 : Inport
  cfblk2 : Outport
  wires:
  cfblk1/1 -> cfblk2/1

== system sampleModel6/cfblk50/cfblk14/cfblk17/cfblk12 ==
  cfblk1 : Inport
  cfblk2 : Outport
  wires:
  cfblk1/1 -> cfblk2/1
